simulink model "robot_wireless_control_system"  (R2020a)
settings: Solver=ode4  StartTime=0.0  StopTime=2.5  FixedStep=5e-4  RelTol=1e-3
undefined symbols (not defined in the file): DiscIntNeverNeededParam
settings Model: Creator=glddy  LastModifiedBy=glddy

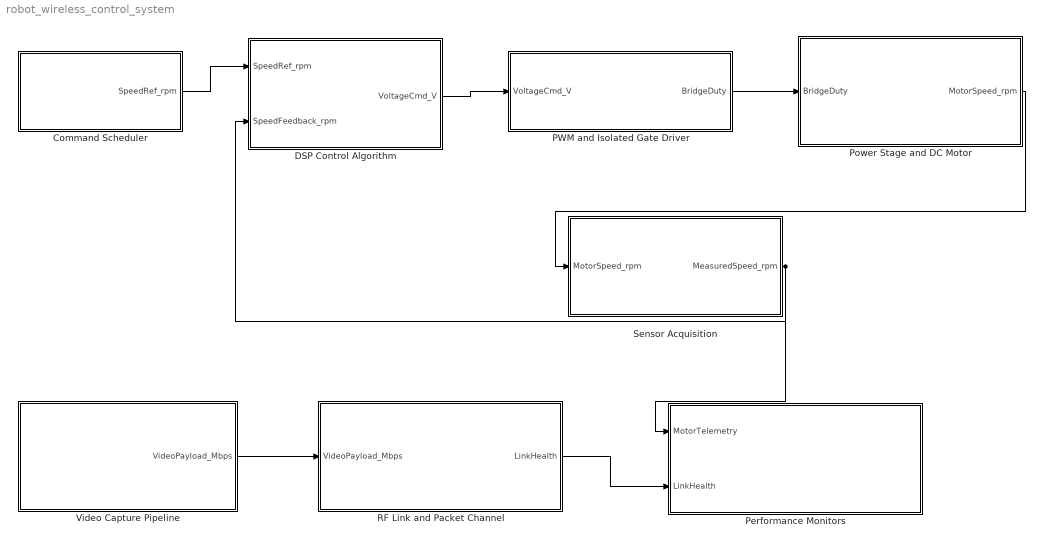
== system robot_wireless_control_system ==
  Command Scheduler : Subsystem
  DSP Control Algorithm : Subsystem
  PWM and Isolated Gate Driver : Subsystem
  Performance Monitors : Subsystem
  Power Stage and DC Motor : Subsystem
  RF Link and Packet Channel : Subsystem
  Sensor Acquisition : Subsystem
  Video Capture Pipeline : Subsystem
  wires:
  Command Scheduler/1(SpeedRef_rpm) -> DSP Control Algorithm/1(SpeedRef_rpm)
  DSP Control Algorithm/1(VoltageCmd_V) -> PWM and Isolated Gate Driver/1(VoltageCmd_V)
  PWM and Isolated Gate Driver/1(BridgeDuty) -> Power Stage and DC Motor/1(BridgeDuty)
  Power Stage and DC Motor/1(MotorSpeed_rpm) -> Sensor Acquisition/1(MotorSpeed_rpm)
  Sensor Acquisition/1(MeasuredSpeed_rpm) -> DSP Control Algorithm/2(SpeedFeedback_rpm), Performance Monitors/1(MotorTelemetry)
  Video Capture Pipeline/1(VideoPayload_Mbps) -> RF Link and Packet Channel/1(VideoPayload_Mbps)
  RF Link and Packet Channel/1(LinkHealth) -> Performance Monitors/2(LinkHealth)

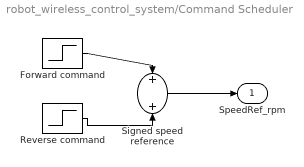
== system robot_wireless_control_system/Command Scheduler ==
  Forward command : Step  Time=0.02  After=600  SampleTime=0
  Reverse command : Step  Time=1.20  After=-1200  SampleTime=0
  Signed speed reference : Sum
  SpeedRef_rpm : Outport
  wires:
  Forward command/1 -> Signed speed reference/1
  Reverse command/1 -> Signed speed reference/2
  Signed speed reference/1 -> SpeedRef_rpm/1

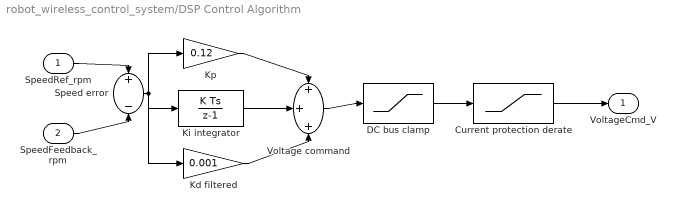
== system robot_wireless_control_system/DSP Control Algorithm ==
  SpeedRef_rpm : Inport
  SpeedFeedback_rpm : Inport  Port=2
  Current protection derate : Saturate  UpperLimit=22  LowerLimit=-22
  DC bus clamp : Saturate  UpperLimit=24  LowerLimit=-24
  Kd filtered : Gain  Gain=0.001
  Ki integrator : DiscreteIntegrator  gainval=3.2  SampleTime=5e-4  ICPrevOutput=DiscIntNeverNeededParam  ICPrevScaledInput=DiscIntNeverNeededParam
  Kp : Gain  Gain=0.12
  Speed error : Sum  Inputs=+-
  Voltage command : Sum  Inputs=+++
  VoltageCmd_V : Outport
  wires:
  SpeedRef_rpm/1 -> Speed error/1
  SpeedFeedback_rpm/1 -> Speed error/2
  Speed error/1 -> Kp/1, Ki integrator/1, Kd filtered/1
  Kp/1 -> Voltage command/1
  Ki integrator/1 -> Voltage command/2
  Kd filtered/1 -> Voltage command/3
  Voltage command/1 -> DC bus clamp/1
  DC bus clamp/1 -> Current protection derate/1
  Current protection derate/1 -> VoltageCmd_V/1

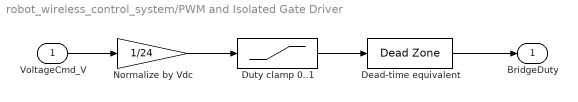
== system robot_wireless_control_system/PWM and Isolated Gate Driver ==
  VoltageCmd_V : Inport
  Dead-time equivalent : DeadZone  LowerValue=-0.02  UpperValue=0.02  SaturateOnIntegerOverflow=on
  Duty clamp 0..1 : Saturate  UpperLimit=1  LowerLimit=-1
  Normalize by Vdc : Gain  Gain=1/24
  BridgeDuty : Outport
  wires:
  VoltageCmd_V/1 -> Normalize by Vdc/1
  Normalize by Vdc/1 -> Duty clamp 0..1/1
  Duty clamp 0..1/1 -> Dead-time equivalent/1
  Dead-time equivalent/1 -> BridgeDuty/1

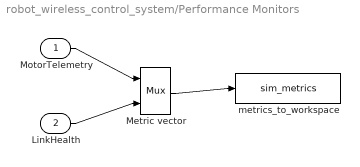
== system robot_wireless_control_system/Performance Monitors ==
  MotorTelemetry : Inport
  LinkHealth : Inport  Port=2
  Metric vector : Mux  Inputs=2
  metrics_to_workspace : ToWorkspace  VariableName=sim_metrics  SaveFormat=Timeseries  SampleTime=-1
  wires:
  MotorTelemetry/1 -> Metric vector/1
  LinkHealth/1 -> Metric vector/2
  Metric vector/1 -> metrics_to_workspace/1

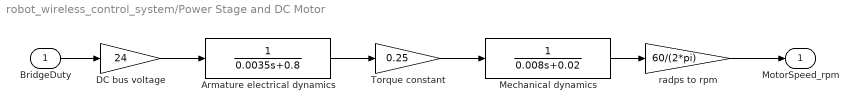
== system robot_wireless_control_system/Power Stage and DC Motor ==
  BridgeDuty : Inport
  Armature electrical dynamics : TransferFcn  Denominator=[0.0035 0.8]
  DC bus voltage : Gain  Gain=24
  Mechanical dynamics : TransferFcn  Denominator=[0.008 0.02]
  Torque constant : Gain  Gain=0.25
  radps to rpm : Gain  Gain=60/(2*pi)
  MotorSpeed_rpm : Outport
  wires:
  BridgeDuty/1 -> DC bus voltage/1
  DC bus voltage/1 -> Armature electrical dynamics/1
  Armature electrical dynamics/1 -> Torque constant/1
  Torque constant/1 -> Mechanical dynamics/1
  Mechanical dynamics/1 -> radps to rpm/1
  radps to rpm/1 -> MotorSpeed_rpm/1

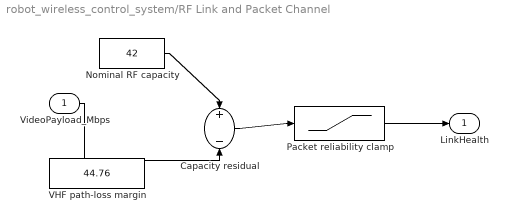
== system robot_wireless_control_system/RF Link and Packet Channel ==
  VideoPayload_Mbps : Inport
  Capacity residual : Sum  Inputs=+-
  Nominal RF capacity : Constant  Value=42
  Packet reliability clamp : Saturate  UpperLimit=1  LowerLimit=0
  VHF path-loss margin : Constant  Value=44.76
  LinkHealth : Outport
  wires:
  Nominal RF capacity/1 -> Capacity residual/1
  VideoPayload_Mbps/1 -> Capacity residual/2
  Capacity residual/1 -> Packet reliability clamp/1
  Packet reliability clamp/1 -> LinkHealth/1

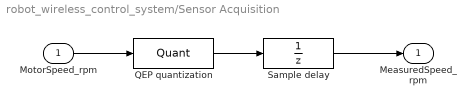
== system robot_wireless_control_system/Sensor Acquisition ==
  MotorSpeed_rpm : Inport
  QEP quantization : Quantizer
  Sample delay : UnitDelay  SampleTime=5e-4  HasFrameUpgradeWarning=on
  MeasuredSpeed_rpm : Outport
  wires:
  MotorSpeed_rpm/1 -> QEP quantization/1
  QEP quantization/1 -> Sample delay/1
  Sample delay/1 -> MeasuredSpeed_rpm/1

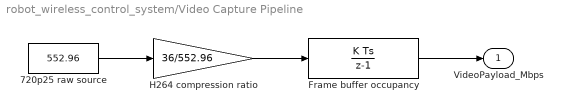
== system robot_wireless_control_system/Video Capture Pipeline ==
  720p25 raw source : Constant  Value=552.96
  Frame buffer occupancy : DiscreteIntegrator  gainval=1  SampleTime=0.04  ICPrevOutput=DiscIntNeverNeededParam  ICPrevScaledInput=DiscIntNeverNeededParam
  H264 compression ratio : Gain  Gain=36/552.96
  VideoPayload_Mbps : Outport
  wires:
  720p25 raw source/1 -> H264 compression ratio/1
  H264 compression ratio/1 -> Frame buffer occupancy/1
  Frame buffer occupancy/1 -> VideoPayload_Mbps/1
